simulink model "fft_sysgen"  (R2014b)
settings: Solver=ode3  SolverMode=SingleTasking  StartTime=0.0  StopTime=Ts*Ns*50  RelTol=1e-3
PreLoadFcn:
  | cd C:\Users\Tim-UML\Documents\GitHub\MA_1\FFT_sysgen_test
StartFcn:
  | cd C:\Users\Tim-UML\Documents\GitHub\MA_1\FFT_sysgen_test
undefined symbols (not defined in the file or in its folder): Ns, Radix, Ts
libraries: xbsIndex_r4 x12, simulink x1, dspxfrm3 x1, commutil2 x1
settings Model: Creator=Tim-UML  LastModifiedBy=Tim-UML

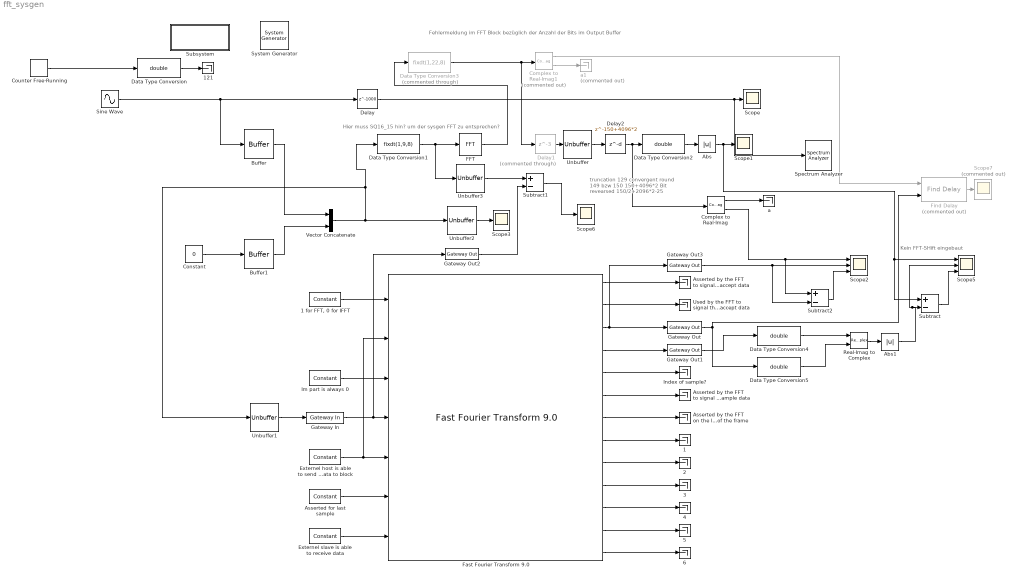
== system fft_sysgen ==
  note: Fehlermeldung im FFT Block bezüglich der Anzahl der Bits im Output Buffer
  note: Hier muss SQ16_15 hin? um der sysgen FFT zu entsprechen?
  note: truncation 129
      | convergent round 149 bzw 150
      | 150+4096*2
      | Bit revearsed 150/2+2096*2-25
  note: Kein FFT-SHift eingebaut
  " System Generator" : xbsIndex_r4/ System Generator  Tag=genX  xilinxfamily=zynq  part=xc7z020  speed=-1  package=clg400  synthesis_tool=Vivado  clock_wrapper=Clock Enables  directory=./netlist  proj_type=Vivado  Synth_file=Vivado Synthesis Defaults  Impl_file=Vivado Implementation Defaults  testbench=off  simulink_period=Ts/2  sysclk_period=10  dcm_input_clock_period=10  incr_netlist=off  trim_vbits=Everywhere in SubSystem  dbl_ovrd=According to Block Masks  core_generation=According to Block Masks  run_coregen=off  deprecated_control=off  eval_field=0  block_type=sysgen
  {1..6,121} (7 alike) : Terminator
  "1 for FFT, 0 for IFFT " : xbsIndex_r4/Constant  const=1  gui_display_data_type=Fixed-point  arith_type=Unsigned  n_bits=1  bin_pt=0  preci_type=Single  exp_width=8  frac_width=24  explicit_period=off  period=1  equ=P=C  opselect=C  inp2=PCIN>>17  opr=+  inp1=P  carry=CIN  dbl_ovrd=off  block_type=constant
  Abs : Abs
  Abs1 : Abs
  "Asserted by the FFT on the last sample of the frame " : Terminator
  "Asserted by the FFT to signal that it is ready to accept data " : Terminator
  "Asserted by the FFT to signal that it is ready to provide sample data " : Terminator
  Asserted for last sample : xbsIndex_r4/Constant  const=0  gui_display_data_type=Boolean  arith_type=Boolean  n_bits=1  bin_pt=0  preci_type=Single  exp_width=8  frac_width=24  explicit_period=off  period=1  equ=P=C  opselect=C  inp2=PCIN>>17  opr=+  inp1=P  carry=CIN  dbl_ovrd=off  block_type=constant
  Buffer : Buffer  N=Ns  TreatMby1Signals=One channel
  Buffer1 : Buffer  N=Ns  TreatMby1Signals=One channel
  Complex to Real-Imag : ComplexToRealImag
  Complex to Real-Imag1 : ComplexToRealImag  Commented=on
  Constant : Constant  Value=0
  Counter Free-Running : simulink/Sources/Counter Free-Running  NumBits=4  tsamp=Ts
  Data Type Conversion : DataTypeConversion  OutDataTypeStr=double
  Data Type Conversion1 : DataTypeConversion  OutDataTypeStr=fixdt(1,9,8)  RndMeth=Convergent  SaturateOnIntegerOverflow=on
  Data Type Conversion2 : DataTypeConversion  OutDataTypeStr=double  RndMeth=Convergent
  Data Type Conversion3 : DataTypeConversion  Commented=through  OutDataTypeStr=fixdt(1,22,8)
  Data Type Conversion4 : DataTypeConversion  OutDataTypeStr=double  RndMeth=Convergent
  Data Type Conversion5 : DataTypeConversion  OutDataTypeStr=double  RndMeth=Convergent
  Delay : Delay  DelayLength=1000  InitialCondition=0
  Delay1 : Delay  Commented=through  DelayLength=3  InitialCondition=0
  Delay2 : Delay  DelayLength=150+4096*2  InitialCondition=0
  Externel host is able to send data to block : xbsIndex_r4/Constant  const=1  gui_display_data_type=Boolean  arith_type=Boolean  n_bits=1  bin_pt=0  preci_type=Single  exp_width=8  frac_width=24  explicit_period=off  period=1  equ=P=C  opselect=C  inp2=PCIN>>17  opr=+  inp1=P  carry=CIN  dbl_ovrd=off  block_type=constant
  "Externel slave is able to receive data " : xbsIndex_r4/Constant  const=1  gui_display_data_type=Boolean  arith_type=Boolean  n_bits=1  bin_pt=0  preci_type=Single  exp_width=8  frac_width=24  explicit_period=off  period=1  equ=P=C  opselect=C  inp2=PCIN>>17  opr=+  inp1=P  carry=CIN  dbl_ovrd=off  block_type=constant
  FFT : dspxfrm3/FFT  CompMethod=Table lookup  TableOpt=NEW  TableOptActive=Speed  BitRevOrder=off  InheritFFTLength=on  FFTLength=64  WrapInput=on  RowConvenienceOn=on  FFTImplementation=Radix-2  SkipNorm=off  firstCoeffDataTypeStr=Inherit: Same word length as input  firstCoeffLastDataTypeStr=Inherit: Same word length as input  outputMode=Binary point scaling  outputWordLength=22  outputFracLength=8  outputDataTypeStr=fixdt(1,22,8)  outputLastDataTypeStr=fixdt(1,22,8)  outputMin=[]  outputMax=[]  roundingMode=Convergent  overflowMode=off
      settings: LockScale=on
  "Fast Fourier Transform 9.0 " : xbsIndex_r4/Fast Fourier Transform 9.0   transform_length=4096  target_clock_frequency=250  target_data_throughput=50  implementation_options=pipelined_streaming_io  run_time_configurable_transform_length=off  phase_factor_width=10  scaling_options=unscaled  rounding_modes=convergent_rounding  aclken=off  aresetn=off  cyclic_prefix_insertion=off  output_ordering=natural_order  throttle_scheme=nonrealtime  xk_index=on  ovflo=off  trim_axipin_name=off  memory_options_data=block_ram  memory_options_phase_factors=block_ram  number_of_stages_using_block_ram_for_data_and_phase_factors=3  memory_options_reorder=block_ram  memory_options_hybrid=off  complex_mult_type=use_mults_resources  butterfly_type=use_luts  channels=1  input_ordering=natural_order  input_width=16  ip_name=Fast Fourier Transform  ip_version=9.0  dsptool_ready=true  ipcore_usecache=true  ipcore_useipmodelcache=true  wrapper_available=true  port_translation_map={ 'aclken' => 'en', 'aresetn' => 'rst'}  data_format=fixed_point  block_type=xfft_v9_0
  Find Delay : commutil2/Find Delay  Commented=on  corrLength=4096  chgSigOP=off  stopUpdate=off  numConstDelay=3
  Gateway In : xbsIndex_r4/Gateway In  gui_display_data_type=Fixed-point  arith_type="Signed  (2's comp)"  n_bits=9  bin_pt=8  preci_type=Double  exp_width=8  frac_width=24  rows=1  columns=1  quantization="Round  (unbiased: +/- Inf)"  overflow=Saturate  period=Ts/2  UseAsADC=off  ADCChannel='1'  interface=None  automatic_assignment=on  address_offset=hex2dec('00')  intf_description=''  timing_constraint=None  locs_specified=off  LOCs={}  io_standard={}  inherit_from_input=off  hdl_port=on  dbl_ovrd=off  block_type=gatewayin
  Gateway Out : xbsIndex_r4/Gateway Out  inherit_from_input=on  hdl_port=on  rows=1  columns=1  UseAsDAC=off  DACChannel='1'  interface=None  automatic_assignment=on  address_offset=hex2dec('00')  intf_description=''  timing_constraint=None  locs_specified=off  LOCs={}  io_standard={}  block_type=gatewayout
  Gateway Out1 : xbsIndex_r4/Gateway Out  inherit_from_input=on  hdl_port=on  rows=1  columns=1  UseAsDAC=off  DACChannel='1'  interface=None  automatic_assignment=on  address_offset=hex2dec('00')  intf_description=''  timing_constraint=None  locs_specified=off  LOCs={}  io_standard={}  block_type=gatewayout
  Gateway Out2 : xbsIndex_r4/Gateway Out  inherit_from_input=on  hdl_port=off  rows=1  columns=1  UseAsDAC=off  DACChannel='1'  interface=None  automatic_assignment=on  address_offset=hex2dec('00')  intf_description=''  timing_constraint=None  locs_specified=off  LOCs={}  io_standard={}  block_type=gatewayout
  Gateway Out3 : xbsIndex_r4/Gateway Out  inherit_from_input=on  hdl_port=off  rows=1  columns=1  UseAsDAC=off  DACChannel='1'  interface=None  automatic_assignment=on  address_offset=hex2dec('00')  intf_description=''  timing_constraint=None  locs_specified=off  LOCs={}  io_standard={}  block_type=gatewayout
  "Im part is always 0 " : xbsIndex_r4/Constant  const=0  gui_display_data_type=Fixed-point  arith_type=Signed (2's comp)  n_bits=9  bin_pt=8  preci_type=Single  exp_width=8  frac_width=24  explicit_period=off  period=1  equ=P=C  opselect=C  inp2=PCIN>>17  opr=+  inp1=P  carry=CIN  dbl_ovrd=off  block_type=constant
  "Index of sample? " : Terminator
  Real-Imag to Complex : RealImagToComplex
  Scope{,1,3,6} (4 alike) : Scope
      Scope1 settings: MaxDataPoints=Ns*2
      Scope3 settings: SaveName=ScopeData3
      Scope6 settings: SaveName=ScopeData6
  Scope2 : Scope  NumInputPorts=3
      settings: YMin=-5~-5~-5  YMax=5~5~5  SaveName=ScopeData2  MaxDataPoints=2*Ns
  Scope5 : Scope  NumInputPorts=3
      settings: YMin=-5~-5~-5  YMax=5~5~5  SaveName=ScopeData5  MaxDataPoints=2*Ns
  Scope7 : Scope  Commented=on
      settings: SaveName=ScopeData7
  Sine Wave : Sin  SineType=Sample based  Frequency=2*pi/Ts/1000  SampleTime=Ts
  Spectrum Analyzer : SpectrumAnalyzer
  Subsystem : Subsystem  mask(Model Parameters){SampleTime=20e-9, SampleCount=2048}
      mask prompts: SampleTime "Sample Time [s]"; SampleCount "Sample Count"
      mask init:
      | initScript_fft_sysgen
      mask Display: disp('Edit Model\n Parameters')
  Subtract : Sum  Inputs=+-
  Subtract1 : Sum  Inputs=+-
  Subtract2 : Sum  Inputs=+-
  Unbuffer{,1..3} (4 alike) : Unbuffer  SampleBasedProcessing=Same as frame based
  Used by the FFT to signal that it is ready to accept data : Terminator
  Vector Concatenate : Concatenate  Mode=Multidimensional array
  a : Terminator
  a1 : Terminator  Commented=on
  wires:
  Unbuffer/1 -> Delay2/1
  Abs/1 -> Subtract/1, Scope5/1, Scope1/1
  Unbuffer2/1 -> Scope3/1
  Delay/1 -> Spectrum Analyzer/1, Scope/1
  Constant/1 -> Buffer1/1
  Buffer/1 -> Vector Concatenate/1
  Vector Concatenate/1 -> Unbuffer1/1, Data Type Conversion1/1, Unbuffer2/1
  Buffer1/1 -> Vector Concatenate/2
  Unbuffer1/1 -> Gateway In/1
  "1 for FFT, 0 for IFFT "/1 -> "Fast Fourier Transform 9.0 "/1
  Gateway In/1 -> Gateway Out2/1, "Fast Fourier Transform 9.0 "/4
  "Fast Fourier Transform 9.0 "/1 -> "Asserted by the FFT to signal that it is ready to accept data "/1
  "Fast Fourier Transform 9.0 "/3 -> Gateway Out3/1, Gateway Out/1
  Externel host is able to send data to block/1 -> "Fast Fourier Transform 9.0 "/2, "Fast Fourier Transform 9.0 "/5
  "Im part is always 0 "/1 -> "Fast Fourier Transform 9.0 "/3
  Asserted for last sample/1 -> "Fast Fourier Transform 9.0 "/6
  "Externel slave is able to receive data "/1 -> "Fast Fourier Transform 9.0 "/7
  "Fast Fourier Transform 9.0 "/2 -> Used by the FFT to signal that it is ready to accept data/1
  "Fast Fourier Transform 9.0 "/5 -> "Index of sample? "/1
  "Fast Fourier Transform 9.0 "/6 -> "Asserted by the FFT to signal that it is ready to provide sample data "/1
  "Fast Fourier Transform 9.0 "/7 -> "Asserted by the FFT on the last sample of the frame "/1
  "Fast Fourier Transform 9.0 "/8 -> 1/1
  "Fast Fourier Transform 9.0 "/9 -> 2/1
  "Fast Fourier Transform 9.0 "/10 -> 3/1
  "Fast Fourier Transform 9.0 "/11 -> 4/1
  "Fast Fourier Transform 9.0 "/12 -> 5/1
  "Fast Fourier Transform 9.0 "/13 -> 6/1
  Gateway Out1/1 -> Data Type Conversion4/1
  Gateway Out/1 -> Data Type Conversion5/1, Find Delay/2
  Real-Imag to Complex/1 -> Abs1/1
  Delay1/1 -> Unbuffer/1
  Abs1/1 -> Scope5/2, Subtract/2
  FFT/1 -> Data Type Conversion3/1
  Delay2/1 -> Data Type Conversion2/1, Complex to Real-Imag/1
  Subtract/1 -> Scope5/3
  Counter Free-Running/1 -> Data Type Conversion/1
  Data Type Conversion/1 -> 121/1
  Sine Wave/1 -> Buffer/1, Delay/1
  Data Type Conversion1/1 -> Unbuffer3/1, FFT/1
  Unbuffer3/1 -> Subtract1/1
  Gateway Out2/1 -> Subtract1/2
  Subtract1/1 -> Scope6/1
  Data Type Conversion3/1 -> Complex to Real-Imag1/1, Delay1/1
  Data Type Conversion4/1 -> Real-Imag to Complex/1
  Data Type Conversion5/1 -> Real-Imag to Complex/2
  Subtract2/1 -> Scope2/3
  Data Type Conversion2/1 -> Abs/1
  Gateway Out3/1 -> Subtract2/2, Scope2/2
  "Fast Fourier Transform 9.0 "/4 -> Gateway Out1/1
  Find Delay/1 -> Scope7/1
  Complex to Real-Imag1/1 -> Find Delay/1
  Complex to Real-Imag1/2 -> a1/1
  Complex to Real-Imag/1 -> a/1
  Complex to Real-Imag/2 -> Subtract2/1, Scope2/1

== system fft_sysgen/Subsystem ==
